simulink model "smart_grid_fault_detection"  (R2025b)
settings: Solver=FixedStepDiscrete  StartTime=0.0  StopTime=0.3  FixedStep=0.00020833333333333335  RelTol=1e-3
settings Model: Creator=Manish  LastModifiedBy=Manish

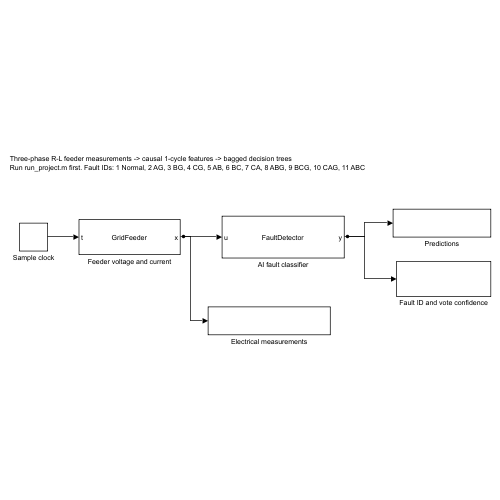
[thumbnail: Simulink's stored preview of the top-level diagram]
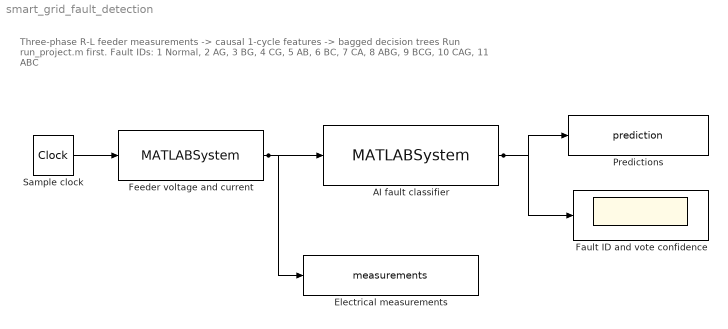
== system smart_grid_fault_detection ==
  note: Three-phase R-L feeder measurements -> causal 1-cycle features -> bagged decision trees
      | Run run_project.m first. Fault IDs: 1 Normal, 2 AG, 3 BG, 4 CG, 5 AB, 6 BC, 7 CA, 8 ABG, 9 BCG, 10 CAG, 11 ABC
  AI fault classifier : MATLABSystem  System=FaultDetector  SimulateUsing=Interpreted execution
      mask Type: FaultDetector
  Electrical measurements : ToWorkspace  VariableName=measurements  SaveFormat=Timeseries  SampleTime=-1
  Fault ID and vote confidence : Scope
  Feeder voltage and current : MATLABSystem  System=GridFeeder  SimulateUsing=Interpreted execution
      mask Type: GridFeeder
  Predictions : ToWorkspace  VariableName=prediction  SaveFormat=Timeseries  SampleTime=-1
  Sample clock : DigitalClock  SampleTime=0.00020833333333333335
  wires:
  Sample clock/1 -> Feeder voltage and current/1
  Feeder voltage and current/1 -> AI fault classifier/1, Electrical measurements/1
  AI fault classifier/1 -> Predictions/1, Fault ID and vote confidence/1
